simulink model "ss_Ref_Discreto_2015"  (Simulink 8.5)
settings: Solver=ode45  SolverMode=SingleTasking  StartTime=0.0  StopTime=10  RelTol=1e-3
values from neighbouring files (symbols this model uses):
  K1 = K(1:end-1)    [Real_Esta_Disc_Ref.m]
  K2 = K(end)    [Real_Esta_Disc_Ref.m]
  Ts = 1    [Real_Esta_Disc_Ref.m]
undefined symbols (not defined in the file or in its folder): Ad, Bd, Cd
settings Model: Creator=Sergio  LastModifiedBy=Sergio  CovMetricSettings=dwe  CovHtmlReporting=off  covSaveCumulativeToWorkspaceVar=off  CovSaveSingleToWorkspaceVar=off  CovExternalEMLEnable=on
settings DataIOCC: LimitDataPoints=off  SaveFormat=Dataset  SignalLoggingSaveFormat=Dataset  ReturnWorkspaceOutputs=on
settings OptimizationCC: ExpressionDepthLimit=128
settings DebuggingCC: UnderspecifiedInitializationDetection=Simplified  MergeDetectMultiDrivingBlocksExec=error  FcnCallInpInsideContextMsg=EnableAllAsError  StateNameClashWarn=none  SFUnexpectedBacktrackingDiag=error  SFNoUnconditionalDefaultTransitionDiag=error
settings HardwareCC: ProdBitPerPointer=64  ProdLargestAtomicFloat=Float  ProdIntDivRoundTo=Zero  ProdEndianess=LittleEndian  ProdHWDeviceType=Specified
settings ModelReferenceCC: PropagateSignalLabelsOutOfModel=on
settings SFSimCC: SimUseLocalCustomCode=on
settings RTWCC: RTWUseLocalCustomCode=on
settings GRTTargetCC: TargetLangStandard=C99 (ISO)  CombineOutputUpdateFcns=on  GRTInterface=off

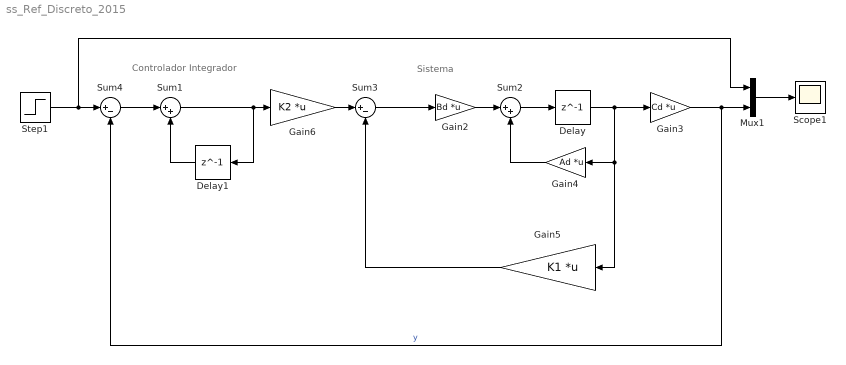
== system ss_Ref_Discreto_2015 ==
  note: Controlador Integrador
  note: Sistema
  Delay : Delay  DelayLength=1  SampleTime=Ts
  Delay1 : Delay  DelayLength=1  SampleTime=Ts
  Gain2 : Gain  Gain=Bd  Multiplication=Matrix(K*u)
  Gain3 : Gain  Gain=Cd  Multiplication=Matrix(K*u)
  Gain4 : Gain  Gain=Ad  Multiplication=Matrix(K*u)
  Gain5 : Gain  Gain=K1  Multiplication=Matrix(K*u)
  Gain6 : Gain  Gain=K2  Multiplication=Matrix(K*u)
  Mux1 : Mux  Inputs=2
  Scope1 : Scope
      settings: TimeRange=auto  ShowLegends=on  MaxDataPoints=5000  SaveToWorkspace=off  YMin=-0.125  YMax=1.125  SampleTime=-1
  Step1 : Step  SampleTime=Ts
  Sum1 : Sum  Inputs=|++
  Sum2 : Sum  Inputs=|++
  Sum3 : Sum  Inputs=|+-
  Sum4 : Sum  Inputs=|+-
  wires:
  Delay/1 -> Gain3/1, Gain5/1, Gain4/1
  Gain4/1 -> Sum2/2
  Sum2/1 -> Delay/1
  Gain2/1 -> Sum2/1
  Sum3/1 -> Gain2/1
  Step1/1 -> Mux1/1, Sum4/1
  Sum4/1 -> Sum1/1
  Sum1/1 -> Delay1/1, Gain6/1
  Gain6/1 -> Sum3/1
  Gain5/1 -> Sum3/2
  Gain3/1 -> Sum4/2, Mux1/2  "y"
  Mux1/1 -> Scope1/1
  Delay1/1 -> Sum1/2
